simulink model "vrplanets"  (Simulink 6.0)
settings: Solver=ode45  StartTime=0.0  StopTime=Inf  RelTol=1e-2
undefined symbols (not defined in the file or in its folder): magnitude
libraries: simulink x3, vrlib x1
settings Model: CovMetricSettings=d  Creator=Dluhos  LastModifiedBy=Houska  ExtModeTrigMode=oneshot  ExtModeArmWhenConnect=off
settings DataIOCC: SaveOutput=off  SaveTime=off  SignalLoggingName=sigsOut
settings OptimizationCC: BlockReduction=off  BooleanDataType=off
settings DebuggingCC: CheckExecutionContextPreStartOutputMsg=on  CheckExecutionContextRuntimeOutputMsg=on  SolverPrmCheckMsg=none
settings HardwareCC: TargetUnknown=on
settings ModelReferenceCC: UpdateModelReferenceTargets=IfOutOfDate
settings GRTTargetCC: LifeSpan=inf
settings SFSimCC: SFSimApplyToAllLibs=on  SFSimBuildMode=Incremental

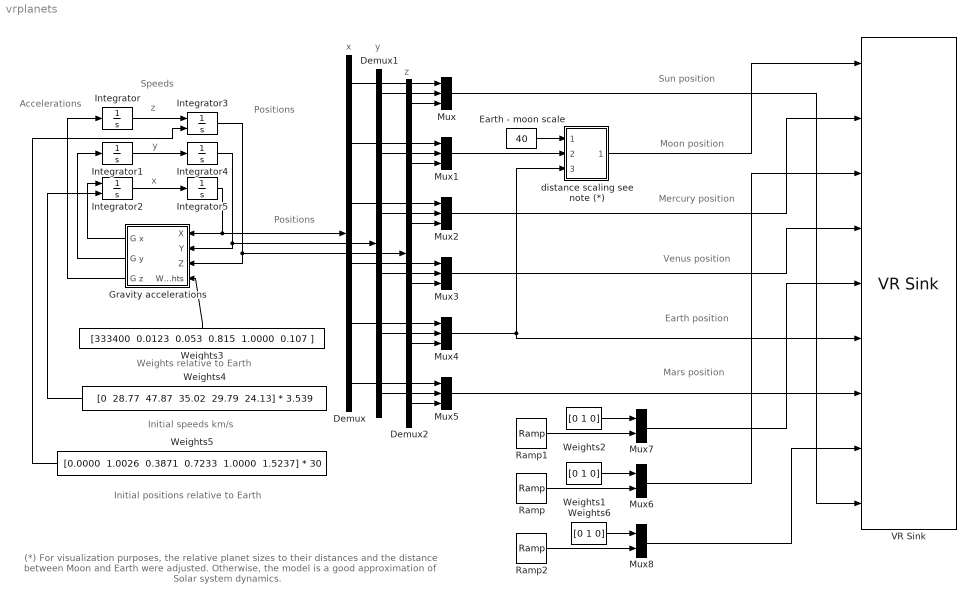
== system vrplanets ==
  note: Positions
  note: Speeds
  note: Accelerations
  note: Weights relative to Earth
  note: Positions
  note: z
  note: y
  note: x
  note: Sun position
  note: Moon position
  note: Mercury position
  note: Venus position
  note: Earth position
  note: Mars position
  note: x
  note: y
  note: z
  note: Initial speeds km/s
  note: Initial positions
      | relative to Earth
  note: (*)  For visualization purposes, the relative planet sizes to their
      | distances and the distance between Moon and Earth were adjusted.
      | Otherwise, the model is a good approximation of Solar system dynamics.
  Demux : Demux  Outputs=6
  Demux1 : Demux  Outputs=6
  Demux2 : Demux  Outputs=6
  Earth - moon scale : Constant  Value=40
  Gravity accelerations : Subsystem  Orientation=left  EnableExecutionContextPropagation=on
  Integrator{,1,4..5} (4 alike) : Integrator  UpperSaturationLimit=Inf  LowerSaturationLimit=-Inf
  Integrator2 : Integrator  InitialConditionSource=external  InitialCondition="[0  0  47.87  35.02  29.79  24.13] * 3.54"  UpperSaturationLimit=Inf  LowerSaturationLimit=-Inf
  Integrator3 : Integrator  InitialConditionSource=external  InitialCondition="[0.0000  1.0200  0.3871  0.7233  1.0000  1.5237] * 30"  UpperSaturationLimit=Inf  LowerSaturationLimit=-Inf
  Mux{,1..5} (6 alike) : Mux  Inputs=3
  Mux6 : Mux  Inputs=2
  Mux7 : Mux  Inputs=2
  Mux8 : Mux  Inputs=2
  Ramp : simulink/Sources/Ramp  slope=11  start=0  X0=0
  Ramp1 : simulink/Sources/Ramp  slope=37  start=0  X0=0
  Ramp2 : simulink/Sources/Ramp  slope=3  start=0  X0=0
  VR Sink : vrlib/VR Sink  SampleTime=0.005  ViewEnable=on  RemoteChange=off  RemoteView=off  FieldsWritten=Moon.translation.3.1.double#Mercury.translation.3.1.double#Venus.rotation.4.1.double#Venus.translation.3.1.double#Earth.rotation.4.1.double#Earth.translation.3.1.double#Mars.translation.3.1.double#Sun.rotation.4.1.double#Sun.translation.3.1.double  WorldFileName=vrplanets.wrl  AutoView=on
  Weights1 : Constant  Value=[0 1 0]
  Weights2 : Constant  Value=[0 1 0]
  Weights3 : Constant  Orientation=up  Value="[333400  0.0123  0.053  0.815  1.0000  0.107 ]"
  Weights4 : Constant  Orientation=left  Value="[0  28.77  47.87  35.02  29.79  24.13] * 3.539"
  Weights5 : Constant  Orientation=left  Value="[0.0000  1.0026  0.3871  0.7233  1.0000  1.5237] * 30"
  Weights6 : Constant  Value=[0 1 0]
  distance scaling see note (*) : Subsystem  EnableExecutionContextPropagation=on
  wires:
  Integrator/1 -> Integrator3/1
  Integrator1/1 -> Integrator4/1
  Integrator2/1 -> Integrator5/1
  Weights3/1 -> Gravity accelerations/4(Weights)
  Gravity accelerations/1(G x) -> Integrator2/1
  Gravity accelerations/2(G y) -> Integrator1/1
  Gravity accelerations/3(G z) -> Integrator/1
  Integrator5/1 -> Gravity accelerations/1(X), Demux/1
  Integrator4/1 -> Gravity accelerations/2(Y), Demux1/1
  Integrator3/1 -> Gravity accelerations/3(Z), Demux2/1
  Weights4/1 -> Integrator2/2
  Weights5/1 -> Integrator3/2
  Demux/1 -> Mux/1
  Demux/2 -> Mux1/1
  Demux/3 -> Mux2/1
  Demux/4 -> Mux3/1
  Demux/5 -> Mux4/1
  Demux/6 -> Mux5/1
  Demux1/1 -> Mux/2
  Demux1/2 -> Mux1/2
  Demux1/3 -> Mux2/2
  Demux1/4 -> Mux3/2
  Demux1/5 -> Mux4/2
  Demux1/6 -> Mux5/2
  Demux2/1 -> Mux/3
  Demux2/2 -> Mux1/3
  Demux2/3 -> Mux2/3
  Demux2/4 -> Mux3/3
  Demux2/5 -> Mux4/3
  Demux2/6 -> Mux5/3
  Earth - moon scale/1 -> distance scaling see note (*)/1(Scale)
  Mux4/1 -> distance scaling see note (*)/3(In2), VR Sink/6
  Weights1/1 -> Mux6/1
  Ramp/1 -> Mux6/2
  Weights2/1 -> Mux7/1
  Ramp1/1 -> Mux7/2
  Mux1/1 -> distance scaling see note (*)/2(In1)
  distance scaling see note (*)/1(Out1) -> VR Sink/1
  Mux2/1 -> VR Sink/2
  Mux6/1 -> VR Sink/3
  Mux3/1 -> VR Sink/4
  Mux7/1 -> VR Sink/5
  Mux5/1 -> VR Sink/7
  Mux/1 -> VR Sink/9
  Weights6/1 -> Mux8/1
  Ramp2/1 -> Mux8/2
  Mux8/1 -> VR Sink/8

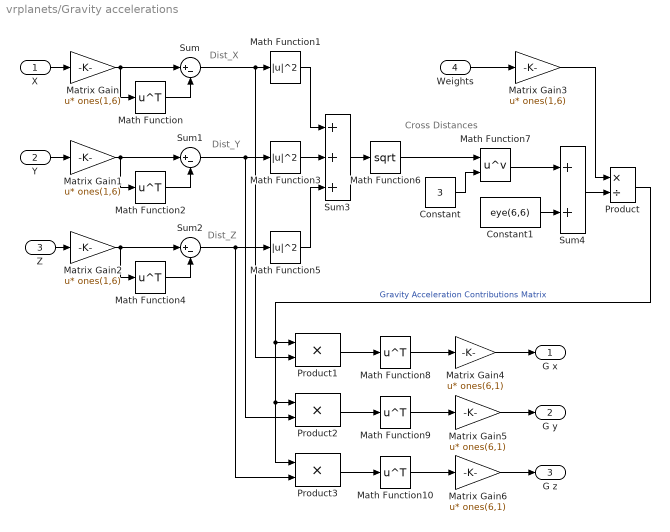
== system vrplanets/Gravity accelerations ==
  note: Dist_Y
  note: Dist_Z
  note: Dist_X
  note: Cross
      | Distances
  X : Inport  LatchInput=off
  Y : Inport  Port=2  LatchInput=off
  Z : Inport  Port=3  LatchInput=off
  Weights : Inport  Port=4  LatchInput=off
  Constant : Constant  Value=3
  Constant1 : Constant  Value=eye(6,6)
  Math Function{,2,4,8..10} (6 alike) : Math  Operator=transpose  SaturateOnIntegerOverflow=on
  Math Function1 : Math  Operator=magnitude^2  SaturateOnIntegerOverflow=on
  Math Function3 : Math  Operator=magnitude^2  SaturateOnIntegerOverflow=on
  Math Function5 : Math  Operator=magnitude^2  SaturateOnIntegerOverflow=on
  Math Function6 : Math  Operator=sqrt  SaturateOnIntegerOverflow=on
  Math Function7 : Math  Operator=pow  SaturateOnIntegerOverflow=on
  Matrix Gain{,1..3} (4 alike) : Gain  Gain=ones(1,6)  Multiplication=Matrix(u*K)  SaturateOnIntegerOverflow=on
  Matrix Gain4 : Gain  Gain=ones(6,1)  Multiplication=Matrix(u*K)  SaturateOnIntegerOverflow=on
  Matrix Gain5 : Gain  Gain=ones(6,1)  Multiplication=Matrix(u*K)  SaturateOnIntegerOverflow=on
  Matrix Gain6 : Gain  Gain=ones(6,1)  Multiplication=Matrix(u*K)  SaturateOnIntegerOverflow=on
  Product : Product  Inputs=*/  SaturateOnIntegerOverflow=on  InputSameDT=on
  Product1 : Product  SaturateOnIntegerOverflow=on  InputSameDT=on
  Product2 : Product  SaturateOnIntegerOverflow=on  InputSameDT=on
  Product3 : Product  SaturateOnIntegerOverflow=on  InputSameDT=on
  Sum : Sum  Inputs=|+-  SaturateOnIntegerOverflow=on  InputSameDT=on
  Sum1 : Sum  Inputs=|+-  SaturateOnIntegerOverflow=on  InputSameDT=on
  Sum2 : Sum  Inputs=|+-  SaturateOnIntegerOverflow=on  InputSameDT=on
  Sum3 : Sum  Inputs=+++  SaturateOnIntegerOverflow=on  InputSameDT=on
  Sum4 : Sum  SaturateOnIntegerOverflow=on  InputSameDT=on
  G x : Outport
  G y : Outport  Port=2
  G z : Outport  Port=3
  wires:
  X/1 -> Matrix Gain/1
  Y/1 -> Matrix Gain1/1
  Z/1 -> Matrix Gain2/1
  Matrix Gain6/1 -> G z/1
  Matrix Gain5/1 -> G y/1
  Matrix Gain4/1 -> G x/1
  Math Function/1 -> Sum/2
  Sum/1 -> Math Function1/1, Product1/2
  Matrix Gain/1 -> Sum/1, Math Function/1
  Math Function2/1 -> Sum1/2
  Sum1/1 -> Math Function3/1, Product2/2
  Math Function3/1 -> Sum3/2
  Matrix Gain1/1 -> Sum1/1, Math Function2/1
  Math Function4/1 -> Sum2/2
  Sum2/1 -> Math Function5/1, Product3/2
  Math Function5/1 -> Sum3/3
  Matrix Gain2/1 -> Sum2/1, Math Function4/1
  Math Function1/1 -> Sum3/1
  Sum3/1 -> Math Function6/1
  Math Function6/1 -> Math Function7/1
  Constant/1 -> Math Function7/2
  Weights/1 -> Matrix Gain3/1
  Math Function7/1 -> Sum4/1
  Constant1/1 -> Sum4/2
  Sum4/1 -> Product/2
  Matrix Gain3/1 -> Product/1
  Product/1 -> Product1/1, Product2/1, Product3/1  "Gravity Acceleration Contributions Matrix"
  Product1/1 -> Math Function8/1
  Math Function8/1 -> Matrix Gain4/1
  Math Function9/1 -> Matrix Gain5/1
  Product2/1 -> Math Function9/1
  Product3/1 -> Math Function10/1
  Math Function10/1 -> Matrix Gain6/1

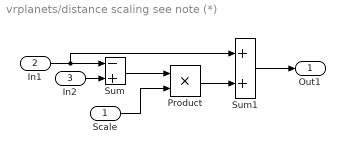
== system vrplanets/distance scaling see note (*) ==
  Scale : Inport  LatchInput=off
  In1 : Inport  Port=2  LatchInput=off
  In2 : Inport  Port=3  LatchInput=off
  Product : Product  SaturateOnIntegerOverflow=on  InputSameDT=on
  Sum : Sum  Inputs=-+  SaturateOnIntegerOverflow=on  InputSameDT=on
  Sum1 : Sum  SaturateOnIntegerOverflow=on  InputSameDT=on
  Out1 : Outport
  wires:
  Sum/1 -> Product/1
  In1/1 -> Sum/1, Sum1/1
  Sum1/1 -> Out1/1
  In2/1 -> Sum/2
  Product/1 -> Sum1/2
  Scale/1 -> Product/2
